simulink library "VehDynaPlayGround"  (R2024b)
settings: Solver=VariableStepAuto  StartTime=0.0  StopTime=10.0  RelTol=1e-3
undefined symbols (not defined in the file or in its folder): A_F, C_af, C_ar, C_d, f, g, h_aero, h_gc, InitialX, InitialY, Iz, lf, lr, m, Nf, Nr, phi, r_stat, r_w, rho, theta, V_wind
libraries: slpidlib x5
(part 3 of 3)

== matlab function VehDynaPlayGround/Model helpers/GetRefference ==
  data: e1 output size=1; de1 output; e2 output; de2 output; e3 output; Vx_reff output; dPsi_des output; X input size=1; Y input double size=1; racetrackwaypoints parameter; Psi input; dPsi input; Vy input; Vx input; phi_ref output
% ******************* GetRefference *********************
%*********************************************************************
% Author: L.Arturo Torres-Romero
% Date: 22-10-2020
% BICYCLE MODEL OF LATERAL VEHICLE DYNAMICS
% Based on Rajamani chapter 2.3 page 30 and  in the next publication with
% the controller
% https://www.researchgate.net/publication/340166902_LATERAL_VEHICLE_DYNAMICS_AND_CONTROLLERS_DESIGN
% This block gets the errors required for the controller of the steering wheel that is based in the error respect the road.
% In this case the road is specified as a list of points (waypoints) in the array racetrackwaypoints
%******************************************************************
%******************* INPUTS DESCRIPTIONS **************************
%******************************************************************
% X:   Global coordinate X of the C.G. of the vehicle 
% Y:   Global coordinate X of the C.G. of the vehicle
% racetrackwaypoints: array with a list of waypoints of the road [X Y]
% Psi: Is the yaw angle respect to the inertial global system
% dPsi: Angular velocity of the yaw angle.
% Vy: Lateral velocity
% Vx: Longitudinal velocity
%******************************************************************
% ******************* OUTPUTS DESCRIPTIONS ************************
%******************************************************************
% e1  : is the lateral position error respect the road.
% de1 : derivative of e1.
% e2  : is the yaw angle error with respect the road. 
% de2 : derivarive of the e2.

function [e1,de1,e2,de2,e3,Vx_reff,dPsi_des,phi_ref] = GetReff(X,Y,racetrackwaypoints, Psi,dPsi, Vy, Vx) 
% Declare msgbox as an extrinsic function
coder.extrinsic('msgbox');
coder.extrinsic('set_param');
coder.extrinsic('uiwait');
coder.extrinsic('movegui');
coder.extrinsic('imread');

persistent lastK;
if isempty(lastK)
    lastK = int32(1); 
end

PQ = [X,Y]; % current Intertial position of vehicle
P = racetrackwaypoints(lastK:end,1:2); % List of waypoints column1 = X coord.  column2 = Y coord. Column 3 = Vx for reference
[k,D] = knnsearch_lib(P,PQ,1); % locate the closest waypoint to the vehicle. k = index, D = distance
k = k(1);

if k > lastK % if we are ahead of the last point searched, then discard the points behind.
    lastK = k-1;
end

% here I take 3 points: the closest, one behind, one in front.
P_road1 = P(k-1,:);
P_road2 = P(k,:);
P_road3 = P(k+1,:);
Vx_reff = racetrackwaypoints(k,3);
Vx_reff = Vx_reff(1);

LookAhead = 5; %how many points ahead to look for the orientation error

if k+LookAhead >= size(P,1)-1 % condition to stop simmulation
    % Display a message dialog

    [img, map] = imread('images/EndFlag.png'); % Cargar la imagen
    h = msgbox('You have arrived!!!', 'Simulation Stop', 'custom', img, map);
    movegui(h, 'northwest');
    % Stop the simulation
    set_param(bdroot, 'SimulationCommand', 'stop');
end

F = atan2( (P(k+LookAhead,2)-P(k,2)),(P(k+LookAhead,1)-P(k,1))); % Obtaining the road orientation
psi_des = F(1);
psi_des = wrapTo2Pi(psi_des);

P_veh = PQ - P_road2;

% Convert from intertial coordinates system to body fixed system. C.G. as
% center and rotated Psi degrees.
M_Rot = [cos(psi_des) -sin(psi_des); sin(psi_des) cos(psi_des)];
P_veh = P_veh*M_Rot;

e1 = P_veh(2); % error e1 that is the y distance from C.G. to desired waypoint from the vehicle reference.
e2 = Psi - psi_des; % error e2 which is the error in the orientation.
e2 = mod(e2 + pi, 2*pi) - pi; % angle adjusted and bounded to -pi to pi.

de1 = Vy + Vx*(e2); % derivative of e1

e3 = P_veh(1); % error e1 that is the x distance from C.G. to desired waypoint from the vehicle reference.

% Obtainig the radius of imaginary circle of the curve
Xc = [P_road1(1);P_road2(1);P_road3(1)];
Yc = [P_road1(2);P_road2(2);P_road3(2)];
[xc,yc,R,a] = circfit(Xc,Yc);
C = [xc yc];
C = (C-P_road2)*M_Rot;
xc = C(1);
yc = C(2);
R = R*sign(yc);


%in streight line, the radius falls into singularity. here is detected
%and solved with a minimum
eval = ~isfinite(R);
if eval
 R = 100000; % in case of NaN define a straight line as an arc of circle of R very big.
end

dPsi_des = Vx/R; % derivative of orientation refference
de2 = dPsi - dPsi_des; % derivative of e2


% sueperelevation of the road or banking
phi_ref = atan(Vx^2/(127*R)); % change for Vx_ref when it is reaady

end

== matlab function VehDynaPlayGround/Control laws/LateralController/DirectLyapunov ==
  data: U output size=1; E input; Vx input; dPsi_des input; C_af parameter; g parameter; C_ar parameter; lf parameter; lr parameter; Iz parameter; m parameter
% ******************* Lateral dynamic controller *********************
%*********************************************************************
% Author: L.Arturo Torres-Romero
% Date: 22-10-2020
% This controller controlls the direction of a car, based in the dynamics
% described  in the next link and using the Direct Lyapunov formulation: 
% https://www.researchgate.net/publication/340166902_LATERAL_VEHICLE_DYNAMICS_AND_CONTROLLERS_DESIGN
%
%ALCALÁ, Eugenio, et al. Comparison of two non-linear model-based control strategies for autonomous vehicles. 
% En 2016 24th Mediterranean Conference on Control and Automation (MED). IEEE, 2016. p. 846-851.
%******************* PARAMETERS DESCRIPTIONS **********************
%******************************************************************
% m: vehicle mass
% g: gravity
% C_af : Cornering  stiffness  of  front  wheels.
% C_ar : Cornering  stiffness  of  rear  wheels.
% lf : distance fron the center of gravity to the front wheel axis.
% lr : distance fron the center of gravity to the rear wheel axis.
% Iz : this is the momentum of inertia of the vehicle respect the z axis.
%******************************************************************
%******************* INPUTS DESCRIPTIONS **************************
%******************************************************************
% E:   (column vector)[e1;de1;e2;de2] states of the state space of 
%       the system that includes the errors as follows:
%      e1  : is the lateral position error respect the road.
%      de1 : derivative of e1.
%      e2  : is the yaw angle error with respect the road. 
%      de2 : derivarive of the e2.
% Vx: Logitudinal velocity.

%******************************************************************
% ******************* OUTPUTS DESCRIPTIONS ************************
%******************************************************************
% U: control coutput in radians. Angle of the frontal wheels respect to the
%    longitudinal axis
% isCtrl: when true means that the matrix Mc has full rank, and hence, the
%         system is controllable
%******************************************************************

function U = DirectLyapunovCtrl(E, Vx,dPsi_des, C_af, g, C_ar, lf, lr, Iz, m) % pd polos deseados

psi_e = E(3);
y_e = E(1);
L = lf+lr;
k2 = 1.1;
k3 = 3;

dPsi_ctrl = dPsi_des -k2*Vx*(sin(psi_e)/psi_e)*y_e - k3*psi_e;

ctrlVal = atan((L*dPsi_ctrl)/Vx);


U = real(ctrlVal);

== matlab function VehDynaPlayGround/Tires/Tyre ModelV1/TireSlip ==
  data: Vx input; s_xf output; w_wf input; r_eff input
%BASED ON
%Rajesh Rajamani, Vehicle Dynamics and Control, Minneapolis, MN, Springer, 2012.
%Chapter 4.1.2
function s_xf = XTireSlip(Vx,w_wf,r_eff) 

if Vx == 0
   s_xf = 0.1 * sign(w_wf);   
else
   s_xf = (r_eff*w_wf -Vx)/abs(Vx); % acceleration
end

if s_xf > 1
   %s_xf = 1; 
end

== matlab function VehDynaPlayGround/Control laws/LateralController/SMC_Alcala/AlcalaSMC ==
  data: U output size=1; E input; Vx input; dPsi_des input; dx_e input; ddPsi_des input; C_af parameter; g parameter; C_ar parameter; lf parameter; lr parameter; Iz parameter; m parameter
% ******************* Lateral dynamic controller *********************
%*********************************************************************
% Author: L.Arturo Torres-Romero
% Date: 22-10-2020
% This controller controlls the direction of a car, based in the dynamics
% described  in the next link and using the Direct Lyapunov formulation: 
% https://www.researchgate.net/publication/340166902_LATERAL_VEHICLE_DYNAMICS_AND_CONTROLLERS_DESIGN
%
%ALCALÁ, Eugenio, et al. Comparison of two non-linear model-based control strategies for autonomous vehicles. 
% En 2016 24th Mediterranean Conference on Control and Automation (MED). IEEE, 2016. p. 846-851.
%******************* PARAMETERS DESCRIPTIONS **********************
%******************************************************************
% m: vehicle mass
% g: gravity
% C_af : Cornering  stiffness  of  front  wheels.
% C_ar : Cornering  stiffness  of  rear  wheels.
% lf : distance fron the center of gravity to the front wheel axis.
% lr : distance fron the center of gravity to the rear wheel axis.
% Iz : this is the momentum of inertia of the vehicle respect the z axis.
%******************************************************************
%******************* INPUTS DESCRIPTIONS **************************
%******************************************************************
% E:   (column vector)[e1;de1;e2;de2] states of the state space of 
%       the system that includes the errors as follows:
%      e1  : is the lateral position error respect the road.
%      de1 : derivative of e1.
%      e2  : is the yaw angle error with respect the road. 
%      de2 : derivarive of the e2.
% Vx: Logitudinal velocity.

%******************************************************************
% ******************* OUTPUTS DESCRIPTIONS ************************
%******************************************************************
% U: control coutput in radians. Angle of the frontal wheels respect to the
%    longitudinal axis
% isCtrl: when true means that the matrix Mc has full rank, and hence, the
%         system is controllable
%******************************************************************

function U = SMC_Ctrl_1(E, Vx,dPsi_des,dx_e,ddPsi_des, C_af, g, C_ar, lf, lr, Iz, m) % pd polos deseados
y_e = E(1);
dy_e = E(2);
psi_e = E(3);
dpsi_e = E(4);
x_e = E(5);


L = lf+lr;
k2 = 2;
k3 = 2.55;
P2 = 3.7;
Q2 = 0.3;

s2 = dy_e +k2*y_e + k3*psi_e;

dPsi_ctrl = dPsi_des + (-P2*s2 -Q2*sign(s2) -k2*dy_e + ddPsi_des*x_e + dPsi_des*dx_e  -Vx*sin(psi_e))/(Vx*sin(psi_e)+k3);

ctrlVal = atan((L*dPsi_ctrl)/Vx);

U = real(ctrlVal);
